simulink model "dof14model_rev"  (R2024a)
settings: Solver=ode4  StartTime=0.0  StopTime=simtime  FixedStep=samtime  RelTol=1e-3
values from neighbouring files (symbols this model uses):
  a = data(n,2)    [main_dof14model.m]
  b = data(n,3)    [main_dof14model.m]
  Csfl = data(n,22)    [main_dof14model.m]
  Csfr = data(n,23)    [main_dof14model.m]
  Csrl = data(n,24)    [main_dof14model.m]
  Csrr = data(n,25)    [main_dof14model.m]
  h = data(n,6)    [main_dof14model.m]
  Ip = data(n,10)    [main_dof14model.m]
  Ir = data(n,11)    [main_dof14model.m]
  Iw = data(n,17)    [main_dof14model.m]
  Jz = data(n,12)    [main_dof14model.m]
  Ksfl = data(n,18)    [main_dof14model.m]
  Ksfr = data(n,19)    [main_dof14model.m]
  Ksrl = data(n,20)    [main_dof14model.m]
  Ksrr = data(n,21)    [main_dof14model.m]
  Ktfl = data(n,28)    [main_dof14model.m]
  Ktfr = data(n,29)    [main_dof14model.m]
  Ktrl = data(n,30)    [main_dof14model.m]
  Ktrr = data(n,31)    [main_dof14model.m]
  Lf = data(n,8)    [main_dof14model.m]
  Lr = data(n,9)    [main_dof14model.m]
  Ms = data(n,1)    [main_dof14model.m]
  mt = data(n,7)    [main_dof14model.m]
  mufl = data(n,13)    [main_dof14model.m]
  mufr = data(n,14)    [main_dof14model.m]
  murl = data(n,15)    [main_dof14model.m]
  murr = data(n,16)    [main_dof14model.m]
  Rw = data(n,27)    [main_dof14model.m]
  wf = data(n,4)    [main_dof14model.m]
  wr = data(n,5)    [main_dof14model.m]
undefined symbols (not defined in the file or in its folder): sigbuilder_block
(part 1 of 2)
settings Model: Creator="Amrik  Singh"  LastModifiedBy=dltkd
settings SolverCC: ZeroCrossAlgorithm=Non-adaptive  AlgebraicLoopSolver=TrustRegion
settings DataIOCC: LimitDataPoints=on  SaveFormat=Array  SignalLoggingSaveFormat=ModelDataLogs  ReturnWorkspaceOutputs=off
settings OptimizationCC: ExpressionDepthLimit=2147483647  InitFltsAndDblsToZero=on  LifeSpan=inf
settings DebuggingCC: UnderspecifiedInitializationDetection=Classic  MergeDetectMultiDrivingBlocksExec=none  SolverPrmCheckMsg=warning  FcnCallInpInsideContextMsg=warning  UnconnectedInputMsg=warning  UnconnectedOutputMsg=warning  UnconnectedLineMsg=warning  StateNameClashWarn=warning  SFUnexpectedBacktrackingDiag=warning  SFNoUnconditionalDefaultTransitionDiag=warning  SFExecutionAtInitializationDiag=none  ArithmeticOperatorsInVariantConditions=warning
settings HardwareCC: ProdBitPerPointer=32  ProdBitPerSizeT=32  ProdBitPerPtrDiffT=32  ProdLargestAtomicFloat=None  ProdIntDivRoundTo=Undefined  ProdEndianess=Unspecified  ProdWordSize=32  ProdHWDeviceType=32-bit Generic
settings ModelReferenceCC: PropagateSignalLabelsOutOfModel=off
settings RTWCC: GPUComputeCapability=3.5
settings CodeAppCC: StateflowObjectComments=on
settings GRTTargetCC: TargetLangStandard=C89/C90 (ANSI)  CombineOutputUpdateFcns=off  GRTInterface=on
settings ConfigComp: CovMetricSettings=dw  CovSaveCumulativeToWorkspaceVar=on  CovSaveSingleToWorkspaceVar=on

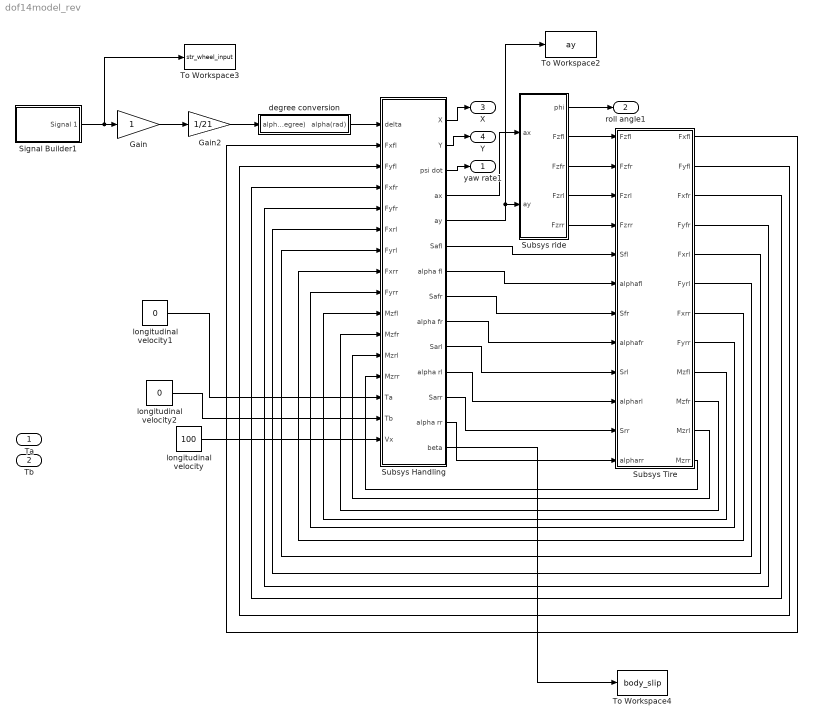
== system dof14model_rev ==
  Ta : Inport
  Tb : Inport  Port=2
  Gain : Gain
  Gain2 : Gain  Gain=1/21
  Signal Builder1 : Subsystem  Tag=STV Subsys  LoadFcn=sigbuilder_block('load');  StartFcn=sigbuilder_block('start');  StopFcn=sigbuilder_block('stop');  ClipboardFcn=sigbuilder_block('clipboard');  mask(Sigbuilder block){tuvar=[0:10]}
      mask help: Sigbuilder GUI
      mask init:
      | if ~strcmp(get_param(bdroot(gcbh),'SimulationStatus'),'stopped') tuvar = sigbuilder_block('maskInit'); end
      settings: CopyFcn=sigbuilder_block('copy');  DeleteFcn=sigbuilder_block('delete');  ModelCloseFcn=sigbuilder_block('modelClose');  PreSaveFcn=sigbuilder_block('preSave');  PauseFcn=sigbuilder_block('pause')  ContinueFcn=sigbuilder_block('continue')  NameChangeFcn=sigbuilder_block('namechange');  OpenFcn=sigbuilder_block('open',[214.5 118.2 550.5 399 ]);  CloseFcn=sigbuilder_block('close');
      mask Display: plot(0, 0, 100, 100,[2, 2, 32, 32, 2], [68, 8, 8, 68, 68],[32, 2], [38, 38], [32, 19, 2],[53, 60, 44], [32, 17, 17, 2],[16, 16, 31, 31]);txt = getActiveGroup(gcbh);text(2, 100, txt,'verticalAlignment', 'top');
  Subsys Handling : Subsystem
  Subsys Tire : Subsystem
  Subsys ride : Subsystem
  To Workspace2 : ToWorkspace  VariableName=ay  SampleTime=-1
      settings: Save2DSignal=2-D array (concatenate along first dimension)
  To Workspace3 : ToWorkspace  VariableName=str_wheel_input  SampleTime=-1
      settings: Save2DSignal=2-D array (concatenate along first dimension)
  To Workspace4 : ToWorkspace  VariableName=body_slip  SampleTime=-1
      settings: Save2DSignal=2-D array (concatenate along first dimension)
  degree conversion : Subsystem
  longitudinal velocity : Constant  Value=100
  longitudinal velocity1 : Constant  Value=0
  longitudinal velocity2 : Constant  Value=0
  yaw rate1 : Outport
  roll angle1 : Outport  Port=2
  X : Outport  Port=3
  Y : Outport  Port=4
  wires:
  Signal Builder1/1(Signal 1) -> To Workspace3/1, Gain/1
  Subsys Handling/2(Y) -> Y/1
  Subsys Tire/5(Fxrl) -> Subsys Handling/6(Fxrl)
  Subsys Handling/1(X) -> X/1
  Subsys Tire/7(Fxrr) -> Subsys Handling/8(Fxrr)
  Subsys ride/3(Fzfr) -> Subsys Tire/2(Fzfr)
  Subsys Tire/4(Fyfr) -> Subsys Handling/5(Fyfr)
  Subsys Handling/5(ay) -> To Workspace2/1, Subsys ride/2(ay)
  Subsys Tire/3(Fxfr) -> Subsys Handling/4(Fxfr)
  Subsys Tire/11(Mzrl) -> Subsys Handling/12(Mzrl)
  Subsys ride/1(phi) -> roll angle1/1
  Subsys ride/2(Fzfl) -> Subsys Tire/1(Fzfl)
  Subsys Tire/12(Mzrr) -> Subsys Handling/13(Mzrr)
  Subsys Tire/6(Fyrl) -> Subsys Handling/7(Fyrl)
  Subsys Handling/11(alpha rl) -> Subsys Tire/10(alpharl)
  Subsys Tire/9(Mzfl) -> Subsys Handling/10(Mzfl)
  Subsys Tire/1(Fxfl) -> Subsys Handling/2(Fxfl)
  Subsys Tire/10(Mzfr) -> Subsys Handling/11(Mzfr)
  Gain2/1 -> degree conversion/1(alpha(degree))
  Subsys Handling/3(psi dot) -> yaw rate1/1
  Subsys ride/5(Fzrr) -> Subsys Tire/4(Fzrr)
  Subsys Handling/6(Safl) -> Subsys Tire/5(Sfl)
  Subsys Tire/2(Fyfl) -> Subsys Handling/3(Fyfl)
  Subsys Handling/13(alpha rr) -> Subsys Tire/12(alpharr)
  Subsys Handling/10(Sarl) -> Subsys Tire/9(Srl)
  Subsys Tire/8(Fyrr) -> Subsys Handling/9(Fyrr)
  longitudinal velocity/1 -> Subsys Handling/16(Vx)
  Gain/1 -> Gain2/1
  Subsys Handling/9(alpha fr) -> Subsys Tire/8(alphafr)
  Subsys Handling/4(ax) -> Subsys ride/1(ax)
  Subsys Handling/8(Safr) -> Subsys Tire/7(Sfr)
  Subsys Handling/12(Sarr) -> Subsys Tire/11(Srr)
  Subsys Handling/7(alpha fl) -> Subsys Tire/6(alphafl)
  Subsys ride/4(Fzrl) -> Subsys Tire/3(Fzrl)
  degree conversion/1(alpha(rad)) -> Subsys Handling/1(delta)
  Subsys Handling/14(beta) -> To Workspace4/1
  longitudinal velocity1/1 -> Subsys Handling/14(Ta)
  longitudinal velocity2/1 -> Subsys Handling/15(Tb)

== system dof14model_rev/Signal Builder1 ==
  Demux : Demux  Tag=STV Demux  Outputs=1
      settings: DisplayOption=none
  FromWs : FromWorkspace  Tag=STV FromWs  VariableName=tuvar
      SigBuilderData=|
      | common.afterFinalStr = 'Extrapolate'
      | common.sampleTime = 0
      | dataSet.timeRange = [0 31]
      | dataSet.name = 'Group 1'
      | sbobj.Name = 'Signal Builder'
      | sbobj.Groups.Name = 'Group 1'
      | sbobj.Groups.Signals.Name = 'Signal 1'
      | sbobj.Groups.Signals.XData = [0 1 31]
      | sbobj.Groups.Signals.YData = [0 0 150]
      | sbobj.Groups.TimeRange = [0 31]
  Signal 1 : Outport  Tag=STV Outport
  wires:
  FromWs/1 -> Demux/1
  Demux/1 -> Signal 1/1

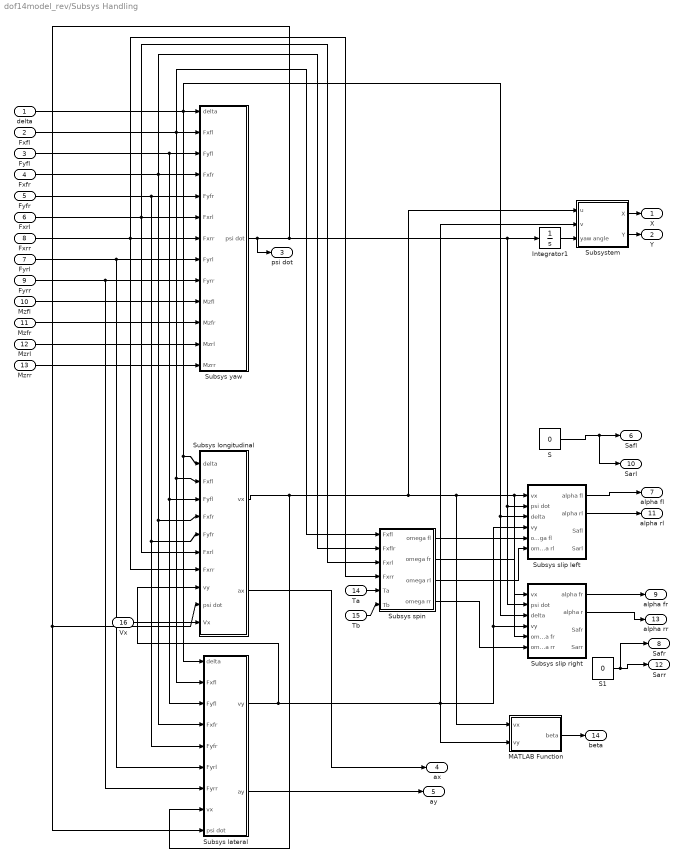
== system dof14model_rev/Subsys Handling ==
  delta : Inport
  Fxfl : Inport  Port=2
  Fyfl : Inport  Port=3
  Fxfr : Inport  Port=4
  Fyfr : Inport  Port=5
  Fxrl : Inport  Port=6
  Fyrl : Inport  Port=7
  Fxrr : Inport  Port=8
  Fyrr : Inport  Port=9
  Mzfl : Inport  Port=10
  Mzfr : Inport  Port=11
  Mzrl : Inport  Port=12
  Mzrr : Inport  Port=13
  Ta : Inport  Port=14
  Tb : Inport  Port=15
  Vx : Inport  Port=16
  Integrator1 : Integrator
  MATLAB Function : MATLAB Function  TreatAsAtomicUnit=on
  S : Constant  Value=0
  S1 : Constant  Value=0
  Subsys lateral : Subsystem
  Subsys longitudinal : Subsystem
  "Subsys slip left " : Subsystem
  Subsys slip right : Subsystem
  Subsys spin : Subsystem
  "Subsys yaw " : Subsystem
  Subsystem : Subsystem
  X : Outport
  Y : Outport  Port=2
  psi dot : Outport  Port=3
  ax : Outport  Port=4
  ay : Outport  Port=5
  Safl : Outport  Port=6
  alpha fl : Outport  Port=7
  Safr : Outport  Port=8
  alpha fr : Outport  Port=9
  Sarl : Outport  Port=10
  alpha rl : Outport  Port=11
  Sarr : Outport  Port=12
  alpha rr : Outport  Port=13
  beta : Outport  Port=14
  wires:
  Subsys lateral/2(ay) -> ay/1
  Subsys longitudinal/2(ax) -> ax/1
  Ta/1 -> Subsys spin/5(Ta)
  Tb/1 -> Subsys spin/6(Tb)
  "Subsys slip left "/1(alpha fl) -> alpha fl/1
  Subsys slip right/1(alpha fr) -> alpha fr/1
  Subsys slip right/2(alpha r) -> alpha rr/1
  Subsys spin/1(omega fl) -> "Subsys slip left "/5(omega fl)
  Subsys spin/4(omega rr) -> Subsys slip right/6(omega rr)
  Subsys longitudinal/1(vx) -> Subsys lateral/8(vx), MATLAB Function/1(vx), "Subsys slip left "/1(vx), Subsys slip right/1(vx), Subsystem/1(u)
  "Subsys slip left "/2(alpha rl) -> alpha rl/1
  delta/1 -> "Subsys yaw "/1(delta), Subsys longitudinal/1(delta), Subsys lateral/1(delta), "Subsys slip left "/3(delta), Subsys slip right/3(delta)
  Fxfl/1 -> "Subsys yaw "/2(Fxfl), Subsys longitudinal/2(Fxfl), Subsys lateral/2(Fxfl), Subsys spin/1(Fxfl)
  Fyfl/1 -> "Subsys yaw "/3(Fyfl), Subsys longitudinal/3(Fyfl), Subsys lateral/3(Fyfl)
  Fxfr/1 -> "Subsys yaw "/4(Fxfr), Subsys longitudinal/4(Fxfr), Subsys lateral/4(Fxfr), Subsys spin/2(Fxflr)
  Fyfr/1 -> "Subsys yaw "/5(Fyfr), Subsys longitudinal/5(Fyfr), Subsys lateral/5(Fyfr)
  Fxrl/1 -> "Subsys yaw "/6(Fxrl), Subsys spin/3(Fxrl), Subsys longitudinal/6(Fxrl)
  Fxrr/1 -> "Subsys yaw "/7(Fxrr), Subsys longitudinal/7(Fxrr), Subsys spin/4(Fxrr)
  Fyrl/1 -> "Subsys yaw "/8(Fyrl), Subsys lateral/6(Fyrl)
  Fyrr/1 -> "Subsys yaw "/9(Fyrr), Subsys lateral/7(Fyrr)
  "Subsys yaw "/1(psi dot) -> Subsys lateral/9("psi dot "), Subsys longitudinal/9("psi dot "), "Subsys slip left "/2(psi dot), Subsys slip right/2(psi dot), Integrator1/1, psi dot/1
  Subsys lateral/1(vy) -> Subsys longitudinal/8(vy), MATLAB Function/2(vy), "Subsys slip left "/4(vy), Subsys slip right/4(vy), Subsystem/2(v)
  Mzfl/1 -> "Subsys yaw "/10(Mzfl)
  Mzrr/1 -> "Subsys yaw "/13(Mzrr)
  Mzrl/1 -> "Subsys yaw "/12(Mzrl)
  Mzfr/1 -> "Subsys yaw "/11(Mzfr)
  Subsys spin/2(omega fr) -> Subsys slip right/5(omega fr)
  Subsys spin/3(omega rl) -> "Subsys slip left "/6(omega rl)
  S/1 -> Safl/1, Sarl/1
  S1/1 -> Sarr/1, Safr/1
  Vx/1 -> Subsys longitudinal/10(Vx)
  Integrator1/1 -> Subsystem/3(yaw angle)
  Subsystem/1(X) -> X/1
  Subsystem/2(Y) -> Y/1
  MATLAB Function/1(beta) -> beta/1

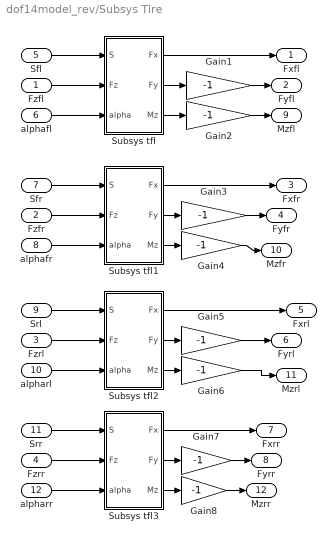
== system dof14model_rev/Subsys Tire ==
  Fzfl : Inport
  Fzfr : Inport  Port=2
  Fzrl : Inport  Port=3
  Fzrr : Inport  Port=4
  Sfl : Inport  Port=5
  alphafl : Inport  Port=6
  Sfr : Inport  Port=7
  alphafr : Inport  Port=8
  Srl : Inport  Port=9
  alpharl : Inport  Port=10
  Srr : Inport  Port=11
  alpharr : Inport  Port=12
  Gain{1..8} (8 alike) : Gain  Gain=-1
  Subsys tfl : Subsystem
  Subsys tfl1 : Subsystem
  Subsys tfl2 : Subsystem
  Subsys tfl3 : Subsystem
  Fxfl : Outport
  Fyfl : Outport  Port=2
  Fxfr : Outport  Port=3
  Fyfr : Outport  Port=4
  Fxrl : Outport  Port=5
  Fyrl : Outport  Port=6
  Fxrr : Outport  Port=7
  Fyrr : Outport  Port=8
  Mzfl : Outport  Port=9
  Mzfr : Outport  Port=10
  Mzrl : Outport  Port=11
  Mzrr : Outport  Port=12
  wires:
  Subsys tfl/1(Fx) -> Fxfl/1
  Subsys tfl/2(Fy) -> Gain1/1
  Subsys tfl/3(Mz) -> Gain2/1
  Sfl/1 -> Subsys tfl/1(S)
  Fzfl/1 -> Subsys tfl/2(Fz)
  alphafl/1 -> Subsys tfl/3(alpha)
  Subsys tfl1/1(Fx) -> Fxfr/1
  Subsys tfl1/2(Fy) -> Gain3/1
  Subsys tfl1/3(Mz) -> Gain4/1
  Sfr/1 -> Subsys tfl1/1(S)
  Fzfr/1 -> Subsys tfl1/2(Fz)
  alphafr/1 -> Subsys tfl1/3(alpha)
  Subsys tfl2/1(Fx) -> Fxrl/1
  Subsys tfl2/2(Fy) -> Gain5/1
  Subsys tfl2/3(Mz) -> Gain6/1
  Srl/1 -> Subsys tfl2/1(S)
  Fzrl/1 -> Subsys tfl2/2(Fz)
  alpharl/1 -> Subsys tfl2/3(alpha)
  Subsys tfl3/1(Fx) -> Fxrr/1
  Subsys tfl3/2(Fy) -> Gain7/1
  Subsys tfl3/3(Mz) -> Gain8/1
  Srr/1 -> Subsys tfl3/1(S)
  Fzrr/1 -> Subsys tfl3/2(Fz)
  alpharr/1 -> Subsys tfl3/3(alpha)
  Gain1/1 -> Fyfl/1
  Gain2/1 -> Mzfl/1
  Gain3/1 -> Fyfr/1
  Gain4/1 -> Mzfr/1
  Gain5/1 -> Fyrl/1
  Gain6/1 -> Mzrl/1
  Gain7/1 -> Fyrr/1
  Gain8/1 -> Mzrr/1

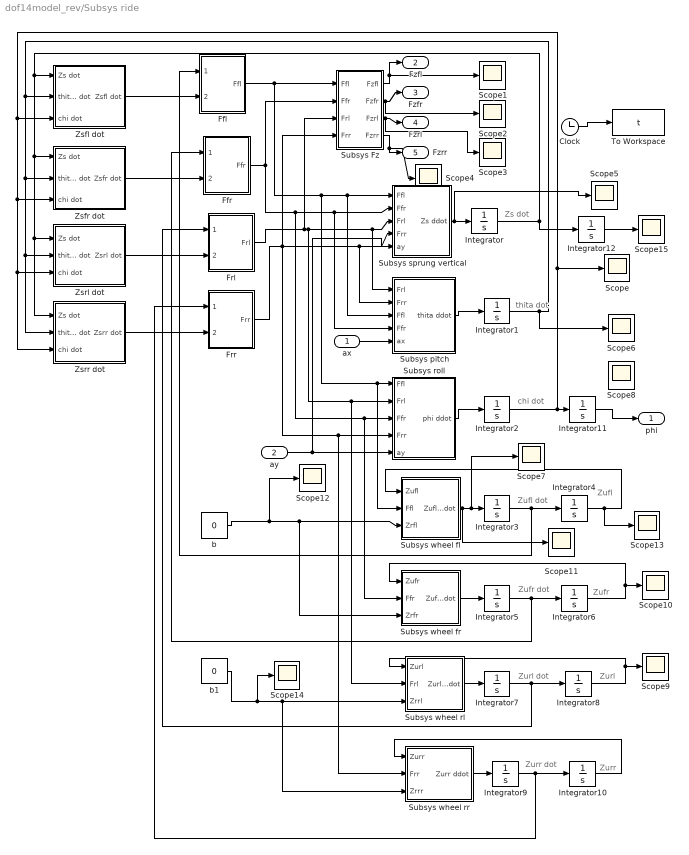
== system dof14model_rev/Subsys ride ==
  note: Zs dot
  note: thita dot
  note: chi dot
  note: Zufl dot
  note: Zufr dot
  note: Zurl dot
  note: Zurr dot
  note: Zufl
  note: Zufr
  note: Zurl
  note: Zurr
  ax : Inport
  ay : Inport  Port=2
  Clock : Clock
  Ffl : Subsystem
  Ffr : Subsystem
  Frl : Subsystem
  Frr : Subsystem
  Integrator{,1..12} (13 alike) : Integrator
  Scope{,1..15} (16 alike) : Scope
  Subsys Fz : Subsystem
  Subsys pitch : Subsystem
  Subsys roll : Subsystem
  Subsys sprung vertical : Subsystem
  Subsys wheel fl : Subsystem
  Subsys wheel fr : Subsystem
  Subsys wheel rl : Subsystem
  Subsys wheel rr : Subsystem
  To Workspace : ToWorkspace  VariableName=t  SampleTime=-1
  Zsfl dot : Subsystem
  Zsfr dot : Subsystem
  Zsrl dot : Subsystem
  Zsrr dot : Subsystem
  b : Constant  Value=0
  b1 : Constant  Value=0
  phi : Outport
  Fzfl : Outport  Port=2
  Fzfr : Outport  Port=3
  Fzrl : Outport  Port=4
  Fzrr : Outport  Port=5
  wires:
  Ffl/1(Ffl) -> Subsys sprung vertical/1(Ffl), Subsys pitch/3(Ffl), Subsys wheel fl/2(Ffl), Subsys roll/1(Ffl), Subsys Fz/1(Ffl)
  Ffr/1(Ffr) -> Subsys sprung vertical/2(Ffr), Subsys pitch/4(Ffr), Subsys wheel fr/2(Ffr), Subsys roll/3(Ffr), Subsys Fz/2(Ffr)
  Frl/1(Frl) -> Subsys sprung vertical/3(Frl), Subsys pitch/1(Frl), Subsys wheel rl/2(Frl), Subsys roll/2(Frl), Subsys Fz/3(Frl)
  Frr/1(Frr) -> Subsys sprung vertical/4(Frr), Subsys pitch/2(Frr), Subsys wheel rr/2(Frr), Subsys roll/4(Frr), Subsys Fz/4(Frr)
  Subsys sprung vertical/1(Zs ddot) -> Integrator/1, Scope5/1
  Integrator/1 -> Zsrr dot/1(Zs dot), Zsrl dot/1(Zs dot), Zsfr dot/1(Zs dot), Zsfl dot/1(Zs dot), Integrator12/1
  Zsfr dot/1(Zsfr dot) -> Ffr/2(Zsfr dot)
  Zsfl dot/1(Zsfl dot) -> Ffl/2(Zsfl dot)
  Zsrl dot/1(Zsrl dot) -> Frl/2(Zsrl dot)
  Zsrr dot/1(Zsrr dot) -> Frr/2(Zsrr dot)
  Subsys pitch/1(thita ddot) -> Integrator1/1
  Subsys roll/1(phi ddot) -> Integrator2/1
  Integrator2/1 -> Zsrr dot/3(chi dot), Zsrl dot/3(chi dot), Zsfr dot/3(chi dot), Zsfl dot/3(chi dot), Scope/1, Integrator11/1
  Subsys wheel fl/1(Zufl ddot) -> Integrator3/1, Scope7/1, Scope11/1
  Integrator3/1 -> Integrator4/1, Ffl/1(Zufl dot)
  Subsys wheel fr/1(Zufr ddot) -> Integrator5/1
  Integrator5/1 -> Integrator6/1, Ffr/1(Zufr dot)
  Subsys wheel rl/1(Zurl ddot) -> Integrator7/1
  Integrator7/1 -> Integrator8/1, Frl/1(Zurl dot)
  Subsys wheel rr/1(Zurr ddot) -> Integrator9/1
  Integrator9/1 -> Integrator10/1, Frr/1(Zurr dot)
  Integrator4/1 -> Subsys wheel fl/1(Zufl), Scope13/1
  Integrator6/1 -> Subsys wheel fr/1(Zufr), Scope10/1
  Integrator8/1 -> Scope9/1, Subsys wheel rl/1(Zurl)
  Integrator10/1 -> Subsys wheel rr/1(Zurr)
  Clock/1 -> To Workspace/1
  Integrator1/1 -> Zsrr dot/2(thita dot), Zsrl dot/2(thita dot), Zsfr dot/2(thita dot), Zsfl dot/2(thita dot), Scope6/1
  Subsys Fz/1(Fzfl) -> Fzfl/1, Scope1/1
  Subsys Fz/2(Fzfr) -> Fzfr/1, Scope2/1
  Subsys Fz/3(Fzrl) -> Fzrl/1, Scope3/1
  Subsys Fz/4(Fzrr) -> Fzrr/1, Scope4/1
  b/1 -> Subsys wheel fl/3(Zrfl), Subsys wheel fr/3(Zrfr), Scope12/1
  b1/1 -> Subsys wheel rl/3(Zrrl), Subsys wheel rr/3(Zrrr), Scope14/1
  ay/1 -> Subsys roll/5(ay), Subsys sprung vertical/5(ay)
  ax/1 -> Subsys pitch/5(ax)
  Integrator11/1 -> phi/1
  Integrator12/1 -> Scope15/1

== system dof14model_rev/degree conversion ==
  alpha(degree) : Inport
  180 degrees : Constant  Value=180
  Divide : Product  Inputs=**/
  pi : Constant  Value=22/7
  alpha(rad) : Outport
  wires:
  alpha(degree)/1 -> Divide/1
  Divide/1 -> alpha(rad)/1
  pi/1 -> Divide/2
  180 degrees/1 -> Divide/3

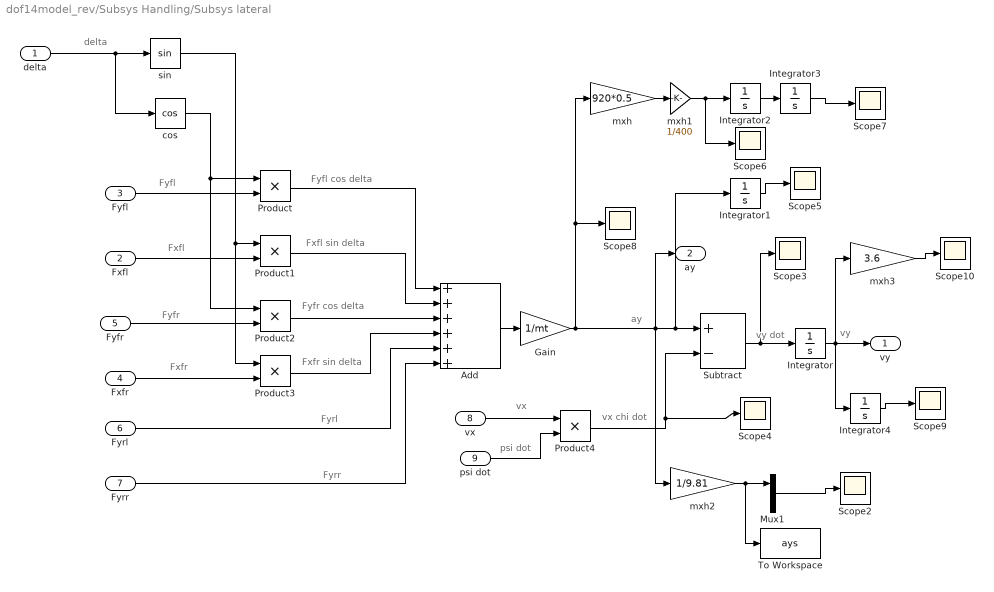
== system dof14model_rev/Subsys Handling/Subsys lateral ==
  note: vy
  note: vy dot
  note: ay
  note: vx
  note: delta
  note: Fyrr
  note: Fyrl
  note: Fxfr
  note: Fyfr
  note: Fxfl
  note: Fyfl
  note: Fyfl cos delta
  note: Fxfl sin delta
  note: Fyfr cos delta
  note: Fxfr sin delta
  note: vx chi dot
  note: psi dot
  delta : Inport
  Fxfl : Inport  Port=2
  Fyfl : Inport  Port=3
  Fxfr : Inport  Port=4
  Fyfr : Inport  Port=5
  Fyrl : Inport  Port=6
  Fyrr : Inport  Port=7
  vx : Inport  Port=8
  "psi dot " : Inport  Port=9
  Add : Sum  Inputs=++++++
  Gain : Gain  Gain=1/mt
  Integrator{,1..4} (5 alike) : Integrator
  Mux1 : Mux  Inputs=2
  Product{,1..4} (5 alike) : Product  RndMeth=Zero
  Scope{2..10} (9 alike) : Scope
  Subtract : Sum  Inputs=+-
  To Workspace : ToWorkspace  VariableName=ays  SampleTime=-1
  cos : Trigonometry  Operator=cos
  mxh : Gain  Gain=920*0.5
  mxh1 : Gain  Gain=1/400
  mxh2 : Gain  Gain=1/9.81
  mxh3 : Gain  Gain=3.6
  sin : Trigonometry
  vy : Outport
  ay : Outport  Port=2
  wires:
  Integrator/1 -> vy/1, Integrator4/1, mxh3/1
  Subtract/1 -> Integrator/1, Scope3/1
  Product4/1 -> Subtract/2, Scope4/1
  Gain/1 -> ay/1, Subtract/1, Integrator1/1, mxh2/1, mxh/1, Scope8/1
  vx/1 -> Product4/1
  Add/1 -> Gain/1
  Fyrr/1 -> Add/6
  Fyrl/1 -> Add/5
  Product3/1 -> Add/4
  Product2/1 -> Add/3
  Product1/1 -> Add/2
  Product/1 -> Add/1
  Fxfr/1 -> Product3/2
  Fyfr/1 -> Product2/2
  Fxfl/1 -> Product1/2
  Fyfl/1 -> Product/2
  sin/1 -> Product1/1, Product3/1
  cos/1 -> Product2/1, Product/1
  delta/1 -> cos/1, sin/1
  Integrator1/1 -> Scope5/1
  "psi dot "/1 -> Product4/2
  Mux1/1 -> Scope2/1
  mxh/1 -> mxh1/1
  Integrator2/1 -> Integrator3/1
  Integrator3/1 -> Scope7/1
  mxh1/1 -> Scope6/1, Integrator2/1
  Integrator4/1 -> Scope9/1
  mxh2/1 -> Mux1/1, To Workspace/1
  mxh3/1 -> Scope10/1

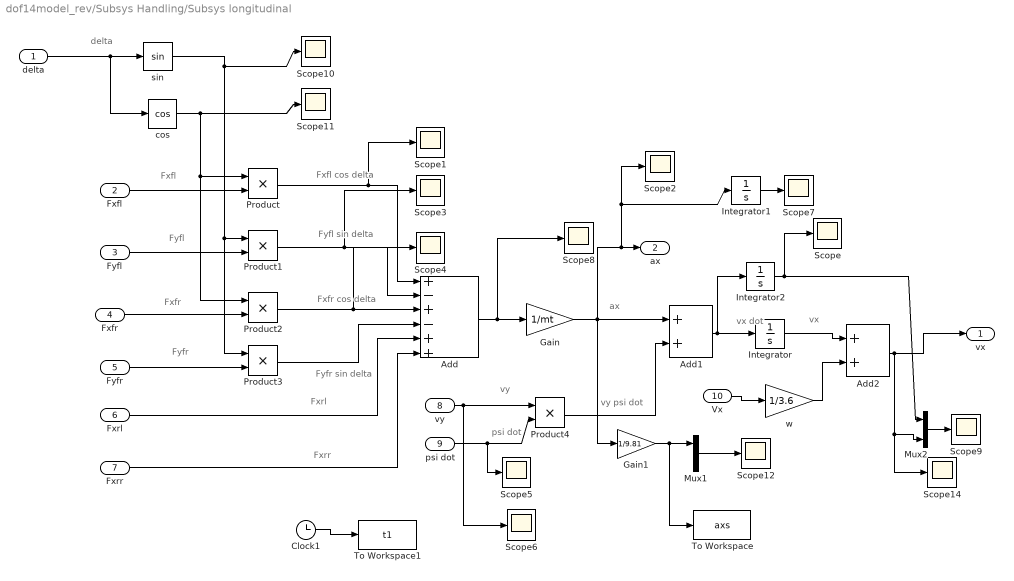
== system dof14model_rev/Subsys Handling/Subsys longitudinal ==
  note: Fxfl
  note: Fyfl
  note: Fxfr
  note: Fyfr
  note: Fxrl
  note: Fxrr
  note: delta
  note: vy
  note: ax
  note: vx dot
  note: vx
  note: Fxfl cos delta
  note: Fyfl sin delta
  note: Fxfr cos delta
  note: Fyfr sin delta
  note: psi dot
  note: vy psi dot
  delta : Inport
  Fxfl : Inport  Port=2
  Fyfl : Inport  Port=3
  Fxfr : Inport  Port=4
  Fyfr : Inport  Port=5
  Fxrl : Inport  Port=6
  Fxrr : Inport  Port=7
  vy : Inport  Port=8
  "psi dot " : Inport  Port=9
  Vx : Inport  Port=10
  Add : Sum  Inputs=+-+-++
  Add1 : Sum
  Add2 : Sum
  Clock1 : Clock
  Gain : Gain  Gain=1/mt
  Gain1 : Gain  Gain=1/9.81
  Integrator : Integrator
  Integrator1 : Integrator
  Integrator2 : Integrator  InitialCondition=50/3.6
  Mux1 : Mux  Inputs=2
  Mux2 : Mux  Inputs=2
  Product{,1..4} (5 alike) : Product  RndMeth=Zero
  Scope{,1..12,14} (14 alike) : Scope
  To Workspace : ToWorkspace  VariableName=axs  SampleTime=-1
  To Workspace1 : ToWorkspace  VariableName=t1  SampleTime=-1
  cos : Trigonometry  Operator=cos
  sin : Trigonometry
  w : Gain  Gain=1/3.6
  vx : Outport
  ax : Outport  Port=2
  wires:
  delta/1 -> sin/1, cos/1
  cos/1 -> Product/1, Product2/1, Scope11/1
  sin/1 -> Product3/1, Product1/1, Scope10/1
  Fxfl/1 -> Product/2
  Fyfl/1 -> Product1/2
  Fxfr/1 -> Product2/2
  Fyfr/1 -> Product3/2
  Product/1 -> Add/1, Scope1/1
  Product1/1 -> Add/2, Scope3/1
  Product2/1 -> Add/3, Scope4/1
  Product3/1 -> Add/4
  Fxrl/1 -> Add/5
  Fxrr/1 -> Add/6
  Add/1 -> Gain/1, Scope8/1
  "psi dot "/1 -> Product4/2, Scope5/1
  vy/1 -> Product4/1, Scope6/1
  Gain/1 -> ax/1, Scope2/1, Integrator1/1, Gain1/1, Add1/1
  Add1/1 -> Integrator/1, Integrator2/1
  Integrator/1 -> Add2/1
  Product4/1 -> Add1/2
  Integrator1/1 -> Scope7/1
  ? -> Mux1/2
  Mux1/1 -> Scope12/1
  Gain1/1 -> Mux1/1, To Workspace/1
  Clock1/1 -> To Workspace1/1
  w/1 -> Add2/2
  Add2/1 -> vx/1, Mux2/2, Scope14/1
  Vx/1 -> w/1
  Mux2/1 -> Scope9/1
  Integrator2/1 -> Mux2/1, Scope/1

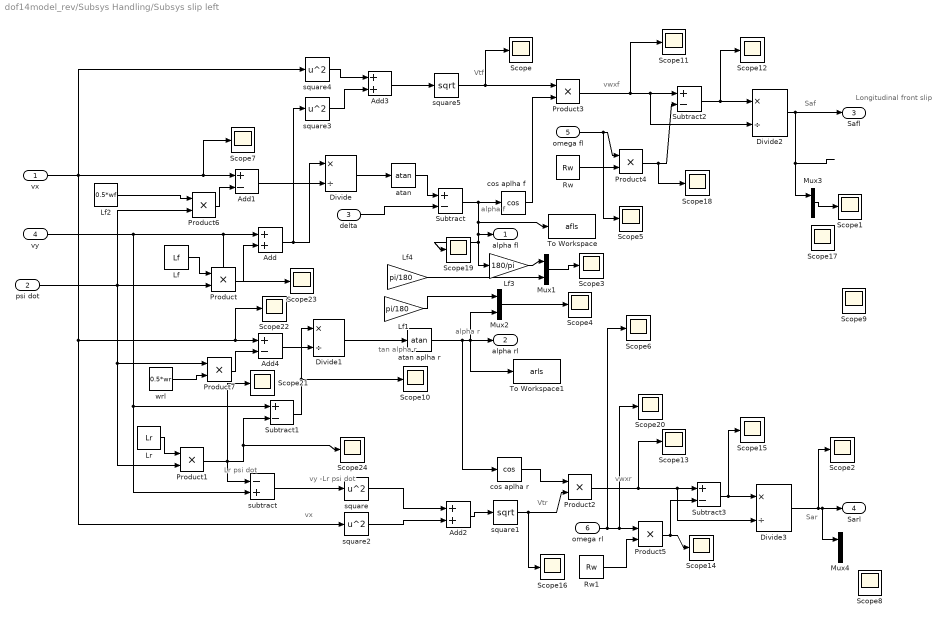
== system dof14model_rev/Subsys Handling/Subsys slip left  ==
  note: tan alpha r
  note: alpha r
  note: Lr psi dot
  note: vx
  note: vy -Lr psi dot
  note: Vtr
  note: alpha f
  note: vwxr
  note: Vtf
  note: vwxf
  note: Saf
  note: Longitudinal front slip
  note: Sar
  vx : Inport
  psi dot : Inport  Port=2
  delta : Inport  Port=3
  vy : Inport  Port=4
  omega fl : Inport  Port=5
  omega rl : Inport  Port=6
  Add : Sum
  Add1 : Sum  Inputs=+-
  Add2 : Sum
  Add3 : Sum
  Add4 : Sum  Inputs=+-
  Divide{,1..3} (4 alike) : Product  Inputs=*/
  Lf : Constant  Value=Lf
  Lf1 : Gain  Gain=pi/180
  Lf2 : Constant  Value=0.5*wf
  Lf3 : Gain  Gain=180/pi
  Lf4 : Gain  Gain=pi/180
  Lr : Constant  Value=Lr
  Mux{1..4} (4 alike) : Mux  Inputs=2
  Product{,1..7} (8 alike) : Product  RndMeth=Zero
  Rw : Constant  Value=Rw
  Rw1 : Constant  Value=Rw
  Scope{,1..24} (25 alike) : Scope
  Subtract{,1..3} (4 alike) : Sum  Inputs=+-
  To Workspace : ToWorkspace  VariableName=afls  SampleTime=-1
  To Workspace1 : ToWorkspace  VariableName=arls  SampleTime=-1
  "atan " : Trigonometry  Operator=atan
  atan aplha r : Trigonometry  Operator=atan
  cos aplha f : Trigonometry  Operator=cos
  cos aplha r : Trigonometry  Operator=cos
  square{,2..4} (4 alike) : Math  Operator=square  SignedPower=on
  square1 : Math  Operator=sqrt  SignedPower=on
  square5 : Math  Operator=sqrt  SignedPower=on
  subtract : Sum  Inputs=-+
  wrl : Constant  Value=0.5*wr
  alpha fl : Outport
  alpha rl : Outport  Port=2
  Safl : Outport  Port=3
  Sarl : Outport  Port=4
  wires:
  Lf/1 -> Product/1
  psi dot/1 -> Product/2, Product6/2, Product1/2, Product7/1
  Add/1 -> Divide/1, square3/1
  delta/1 -> Subtract/2
  vx/1 -> square4/1, Add1/1, Scope7/1, square2/1, Add4/1, Scope22/1
  Product/1 -> Add/2
  vy/1 -> Subtract1/1, subtract/2, Add/1, Scope23/1
  Divide/1 -> "atan "/1
  "atan "/1 -> Subtract/1
  Subtract1/1 -> Divide1/1, Scope10/1
  Lr/1 -> Product1/1
  Product1/1 -> subtract/1, Scope21/1, Subtract1/2, Scope24/1
  Divide1/1 -> atan aplha r/1
  atan aplha r/1 -> cos aplha r/1, alpha rl/1, Mux2/2, To Workspace1/1
  subtract/1 -> square/1
  square/1 -> Add2/1
  square2/1 -> Add2/2
  Add2/1 -> square1/1
  square1/1 -> Product2/2, Scope16/1
  cos aplha r/1 -> Product2/1
  Product2/1 -> Scope13/1, Subtract3/1, Divide3/2
  square4/1 -> Add3/1
  square3/1 -> Add3/2
  Add3/1 -> square5/1
  Subtract/1 -> cos aplha f/1, alpha fl/1, Lf3/1, Scope19/1, To Workspace/1
  square5/1 -> Product3/1, Scope/1
  cos aplha f/1 -> Product3/2
  Product3/1 -> Subtract2/1, Divide2/2, Scope11/1
  omega fl/1 -> Product4/1, Scope5/1
  Rw/1 -> Product4/2
  Product4/1 -> Subtract2/2, Scope18/1
  Subtract2/1 -> Divide2/1, Scope12/1
  Divide2/1 -> Safl/1, Mux3/1
  omega rl/1 -> Scope6/1, Product5/1, Scope20/1
  Rw1/1 -> Product5/2
  Product5/1 -> Scope14/1, Subtract3/2
  Subtract3/1 -> Divide3/1, Scope15/1
  Divide3/1 -> Sarl/1, Mux4/1, Scope2/1
  ? -> Lf4/1
  Mux1/1 -> Scope3/1
  Lf4/1 -> Mux1/2
  ? -> Lf1/1
  Mux2/1 -> Scope4/1
  Lf1/1 -> Mux2/1
  ? -> Mux3/2, Scope17/1
  Mux3/1 -> Scope1/1
  ? -> Scope9/1
  Add1/1 -> Divide/2
  Product6/1 -> Add1/2
  Lf2/1 -> Product6/1
  wrl/1 -> Product7/2
  Add4/1 -> Divide1/2
  Product7/1 -> Add4/2
  ? -> Scope8/1
  Lf3/1 -> Mux1/1

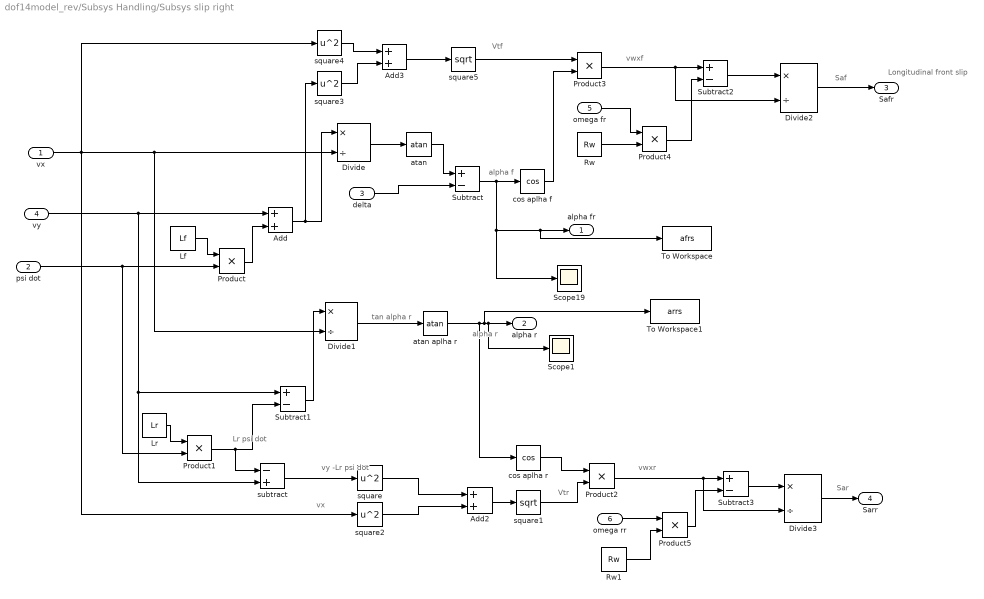
== system dof14model_rev/Subsys Handling/Subsys slip right ==
  note: Sar
  note: Longitudinal front slip
  note: Saf
  note: vwxf
  note: Vtf
  note: vwxr
  note: alpha f
  note: Vtr
  note: vy -Lr psi dot
  note: vx
  note: Lr psi dot
  note: alpha r
  note: tan alpha r
  vx : Inport
  psi dot : Inport  Port=2
  delta : Inport  Port=3
  vy : Inport  Port=4
  omega fr : Inport  Port=5
  omega rr : Inport  Port=6
  Add : Sum
  Add2 : Sum
  Add3 : Sum
  Divide{,1..3} (4 alike) : Product  Inputs=*/
  Lf : Constant  Value=Lf
  Lr : Constant  Value=Lr
  Product{,1..5} (6 alike) : Product  RndMeth=Zero
  Rw : Constant  Value=Rw
  Rw1 : Constant  Value=Rw
  Scope1 : Scope
  Scope19 : Scope
  Subtract{,1..3} (4 alike) : Sum  Inputs=+-
  To Workspace : ToWorkspace  VariableName=afrs  SampleTime=-1
  To Workspace1 : ToWorkspace  VariableName=arrs  SampleTime=-1
  "atan " : Trigonometry  Operator=atan
  atan aplha r : Trigonometry  Operator=atan
  cos aplha f : Trigonometry  Operator=cos
  cos aplha r : Trigonometry  Operator=cos
  square{,2..4} (4 alike) : Math  Operator=square  SignedPower=on
  square1 : Math  Operator=sqrt  SignedPower=on
  square5 : Math  Operator=sqrt  SignedPower=on
  subtract : Sum  Inputs=-+
  alpha fr : Outport
  alpha r : Outport  Port=2
  Safr : Outport  Port=3
  Sarr : Outport  Port=4
  wires:
  Divide3/1 -> Sarr/1
  Subtract3/1 -> Divide3/1
  Product5/1 -> Subtract3/2
  Rw1/1 -> Product5/2
  omega rr/1 -> Product5/1
  Divide2/1 -> Safr/1
  Subtract2/1 -> Divide2/1
  Product4/1 -> Subtract2/2
  Rw/1 -> Product4/2
  omega fr/1 -> Product4/1
  Product3/1 -> Divide2/2, Subtract2/1
  cos aplha f/1 -> Product3/2
  square5/1 -> Product3/1
  Subtract/1 -> cos aplha f/1, Scope19/1, alpha fr/1, To Workspace/1
  Add3/1 -> square5/1
  square3/1 -> Add3/2
  square4/1 -> Add3/1
  Product2/1 -> Divide3/2, Subtract3/1
  cos aplha r/1 -> Product2/1
  square1/1 -> Product2/2
  Add2/1 -> square1/1
  square2/1 -> Add2/2
  square/1 -> Add2/1
  subtract/1 -> square/1
  atan aplha r/1 -> cos aplha r/1, alpha r/1, Scope1/1, To Workspace1/1
  Divide1/1 -> atan aplha r/1
  Product1/1 -> subtract/1, Subtract1/2
  Lr/1 -> Product1/1
  Subtract1/1 -> Divide1/1
  "atan "/1 -> Subtract/1
  Divide/1 -> "atan "/1
  vy/1 -> subtract/2, Subtract1/1, Add/1
  Product/1 -> Add/2
  vx/1 -> square4/1, Divide1/2, Divide/2, square2/1
  delta/1 -> Subtract/2
  Add/1 -> square3/1, Divide/1
  psi dot/1 -> Product1/2, Product/2
  Lf/1 -> Product/1

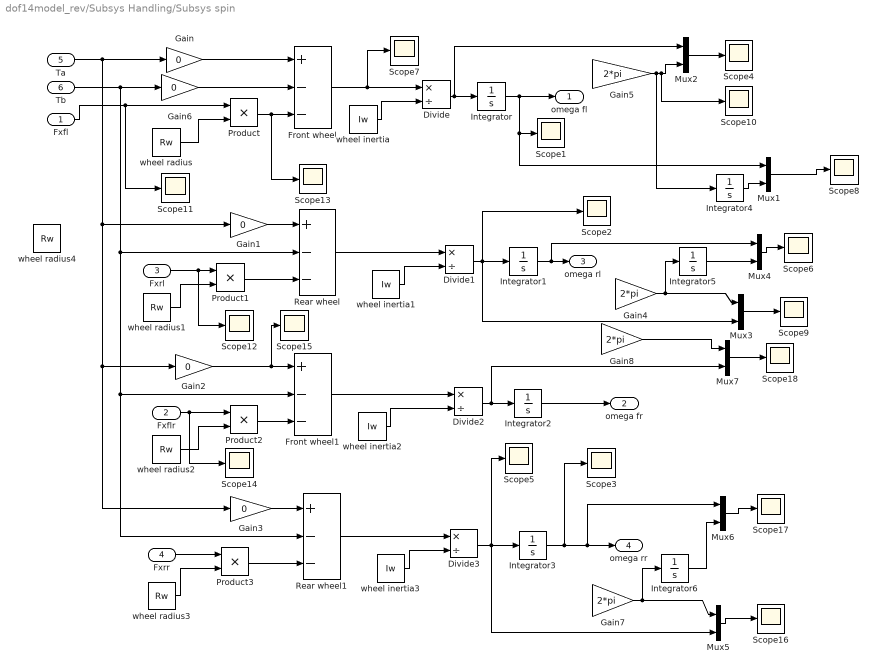
== system dof14model_rev/Subsys Handling/Subsys spin ==
  Fxfl : Inport
  Fxflr : Inport  Port=2
  Fxrl : Inport  Port=3
  Fxrr : Inport  Port=4
  Ta : Inport  Port=5
  Tb : Inport  Port=6
  Divide{,1..3} (4 alike) : Product  Inputs=*/
  Front wheel : Sum  Inputs=+--
  Front wheel1 : Sum  Inputs=+--
  Gain{,1..3,6} (5 alike) : Gain  Gain=0
  Gain{4..5,7..8} (4 alike) : Gain  Gain=2*pi
  Integrator{,1..6} (7 alike) : Integrator
  Mux{1..7} (7 alike) : Mux  Inputs=2
  Product{,1..3} (4 alike) : Product  RndMeth=Zero
  Rear wheel : Sum  Inputs=+--
  Rear wheel1 : Sum  Inputs=+--
  Scope{1..18} (18 alike) : Scope
  wheel inertia{,1..3} (4 alike) : Constant  Value=Iw
  wheel radius{,1..4} (5 alike) : Constant  Value=Rw
  omega fl : Outport
  omega fr : Outport  Port=2
  omega rl : Outport  Port=3
  omega rr : Outport  Port=4
  wires:
  Ta/1 -> Gain/1, Gain1/1, Gain2/1, Gain3/1
  Gain1/1 -> Rear wheel/1
  Gain/1 -> Front wheel/1
  Tb/1 -> Rear wheel/2, Front wheel1/2, Rear wheel1/2, Gain6/1
  Front wheel/1 -> Divide/1, Scope7/1
  Rear wheel/1 -> Divide1/1
  Product1/1 -> Rear wheel/3
  wheel inertia/1 -> Divide/2
  wheel inertia1/1 -> Divide1/2
  Divide/1 -> Integrator/1, Mux2/1
  Divide1/1 -> Integrator1/1, Scope2/1, Mux3/2
  Fxfl/1 -> Product/1, Scope11/1
  Product/1 -> Front wheel/3, Scope13/1
  wheel radius/1 -> Product/2
  Fxrl/1 -> Product1/1, Scope12/1
  wheel radius1/1 -> Product1/2
  Gain2/1 -> Front wheel1/1, Scope15/1
  Front wheel1/1 -> Divide2/1
  wheel inertia2/1 -> Divide2/2
  Fxflr/1 -> Product2/1, Scope14/1
  Product2/1 -> Front wheel1/3
  wheel radius2/1 -> Product2/2
  Gain3/1 -> Rear wheel1/1
  Rear wheel1/1 -> Divide3/1
  Product3/1 -> Rear wheel1/3
  wheel inertia3/1 -> Divide3/2
  Divide3/1 -> Integrator3/1, Scope5/1, Mux5/2
  Fxrr/1 -> Product3/1
  wheel radius3/1 -> Product3/2
  Integrator/1 -> omega fl/1, Scope1/1, Mux1/1
  Integrator1/1 -> omega rl/1, Mux4/1
  Divide2/1 -> Integrator2/1, Mux7/2
  Integrator2/1 -> omega fr/1
  Integrator3/1 -> Scope3/1, omega rr/1, Mux6/1
  Mux1/1 -> Scope8/1
  ? -> Gain5/1
  Gain5/1 -> Integrator4/1, Mux2/2, Scope10/1
  Mux2/1 -> Scope4/1
  Integrator4/1 -> Mux1/2
  Mux3/1 -> Scope9/1
  ? -> Gain4/1
  Gain4/1 -> Mux3/1, Integrator5/1
  Integrator5/1 -> Mux4/2
  Mux4/1 -> Scope6/1
  Gain6/1 -> Front wheel/2
  Mux5/1 -> Scope16/1
  ? -> Gain7/1
  Gain7/1 -> Mux5/1, Integrator6/1
  Integrator6/1 -> Mux6/2
  Mux6/1 -> Scope17/1
  Mux7/1 -> Scope18/1
  Gain8/1 -> Mux7/1
  ? -> Gain8/1

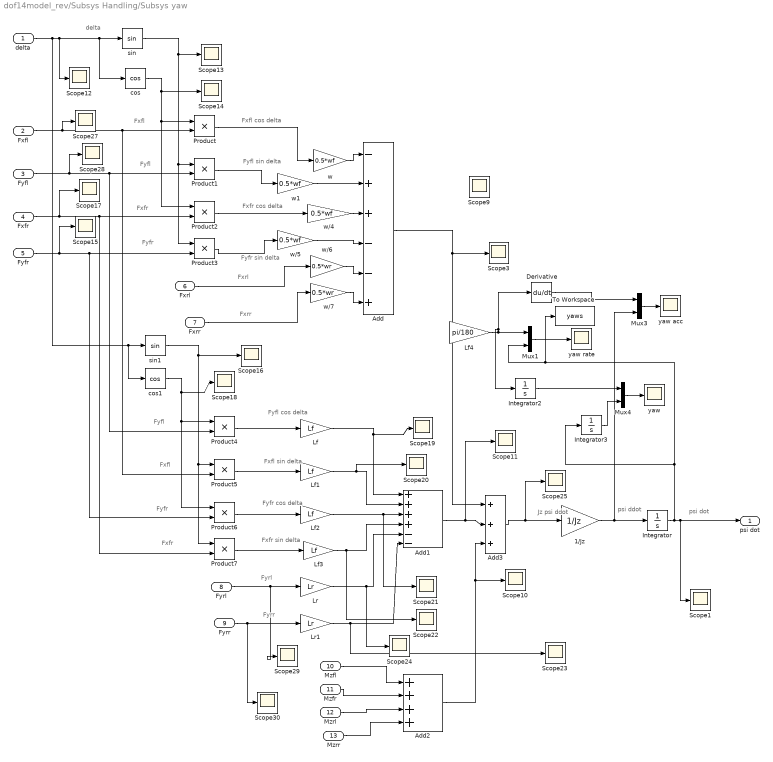
== system dof14model_rev/Subsys Handling/Subsys yaw  ==
  note: Fxfl
  note: Fyfl
  note: Fxfr
  note: Fyfr
  note: Fxrl
  note: Fxrr
  note: delta
  note: Fxfl cos delta
  note: Fyfl sin delta
  note: Fxfr cos delta
  note: Fyfr sin delta
  note: Fyrr
  note: Fyrl
  note: Fxfr
  note: Fyfr
  note: Fxfl
  note: Fyfl
  note: Fyfl cos delta
  note: Fxfl sin delta
  note: Fyfr cos delta
  note: Fxfr sin delta
  note: Jz psi ddot
  note: psi ddot
  note: psi dot
  delta : Inport
  Fxfl : Inport  Port=2
  Fyfl : Inport  Port=3
  Fxfr : Inport  Port=4
  Fyfr : Inport  Port=5
  Fxrl : Inport  Port=6
  Fxrr : Inport  Port=7
  Fyrl : Inport  Port=8
  Fyrr : Inport  Port=9
  Mzfl : Inport  Port=10
  Mzfr : Inport  Port=11
  Mzrl : Inport  Port=12
  Mzrr : Inport  Port=13
  1/Jz : Gain  Gain=1/Jz
  Add : Sum  Inputs=-++--+
  Add1 : Sum  Inputs=++++--
  Add2 : Sum  Inputs=++++
  Add3 : Sum  Inputs=+++
  Derivative : Derivative
  Integrator : Integrator
  Integrator2 : Integrator
  Integrator3 : Integrator
  Lf{,1..3} (4 alike) : Gain  Gain=Lf
  Lf4 : Gain  Gain=pi/180
  Lr : Gain  Gain=Lr
  Lr1 : Gain  Gain=Lr
  Mux1 : Mux  Inputs=2
  Mux3 : Mux  Inputs=2
  Mux4 : Mux  Inputs=2
  Product{,1..7} (8 alike) : Product  RndMeth=Zero
  Scope{1,3,9..25,27..30} (23 alike) : Scope
  To Workspace : ToWorkspace  VariableName=yaws  SampleTime=-1
  cos : Trigonometry  Operator=cos
  cos1 : Trigonometry  Operator=cos
  sin : Trigonometry
  sin1 : Trigonometry
  w : Gain  Gain=0.5*wf
  w/4 : Gain  Gain=0.5*wf
  w/5 : Gain  Gain=0.5*wf
  w/6 : Gain  Gain=0.5*wr
  w/7 : Gain  Gain=0.5*wr
  w1 : Gain  Gain=0.5*wf
  yaw : Scope
  yaw acc : Scope
  yaw rate : Scope
  psi dot : Outport
  wires:
  delta/1 -> sin1/1, cos1/1, sin/1, cos/1, Scope12/1
  cos/1 -> Product/1, Product2/1, Scope14/1
  sin/1 -> Product3/1, Product1/1, Scope13/1
  Fxfl/1 -> Product/2, Product5/2, Scope27/1
  Fyfl/1 -> Product1/2, Product4/2, Scope28/1
  Fxfr/1 -> Product2/2, Product7/2, Scope17/1
  Fyfr/1 -> Product3/2, Product6/2, Scope15/1
  Product2/1 -> w/4/1
  Product3/1 -> w/5/1
  Fxrl/1 -> w/6/1
  Fxrr/1 -> w/7/1
  Product1/1 -> w1/1
  Product/1 -> w/1
  sin1/1 -> Product5/1, Product7/1, Scope16/1
  cos1/1 -> Product6/1, Product4/1, Scope18/1
  Product4/1 -> Lf/1
  Lf/1 -> Add1/1, Scope19/1
  Product5/1 -> Lf1/1
  Product6/1 -> Lf2/1
  Product7/1 -> Lf3/1
  Lf1/1 -> Add1/2, Scope20/1
  Lf2/1 -> Add1/3, Scope21/1
  Lf3/1 -> Add1/4, Scope22/1
  Fyrr/1 -> Lr1/1, Scope30/1
  Lr/1 -> Add1/5, Scope24/1
  Lr1/1 -> Add1/6, Scope23/1
  Add/1 -> Add3/1, Scope3/1
  Fyrl/1 -> Lr/1, Scope29/1
  Integrator/1 -> Integrator3/1, Mux1/2, To Workspace/1, Scope1/1, psi dot/1
  1/Jz/1 -> Integrator/1, Mux3/2
  Add3/1 -> 1/Jz/1, Scope25/1
  Add1/1 -> Scope11/1, Add3/2
  ? -> Lf4/1
  Mux1/1 -> yaw rate/1
  w/1 -> Add/1
  w1/1 -> Add/2
  w/4/1 -> Add/3
  w/5/1 -> Add/4
  w/6/1 -> Add/5
  w/7/1 -> Add/6
  Mzfl/1 -> Add2/1
  Mzfr/1 -> Add2/2
  Add2/1 -> Scope10/1, Add3/3
  Mzrl/1 -> Add2/3
  Mzrr/1 -> Add2/4
  Lf4/1 -> Derivative/1, Integrator2/1, Mux1/1
  Mux3/1 -> yaw acc/1
  Derivative/1 -> Mux3/1
  Integrator2/1 -> Mux4/1
  Integrator3/1 -> Mux4/2
  Mux4/1 -> yaw/1

== system dof14model_rev/Subsys Handling/Subsystem ==
  u : Inport
  v : Inport  Port=2
  yaw angle : Inport  Port=3
  Add : Sum
  Add1 : Sum  Inputs=+-
  Integrator : Integrator
  Integrator1 : Integrator
  Product{,1..3} (4 alike) : Product  RndMeth=Zero
  X1 : Scope
  Y1 : Scope
  cos : Trigonometry  Operator=cos
  cos1 : Trigonometry
  X : Outport
  Y : Outport  Port=2
  wires:
  yaw angle/1 -> cos/1, cos1/1
  u/1 -> Product1/1, Product/1
  cos/1 -> Product1/2, Product3/2
  cos1/1 -> Product2/2, Product/2
  v/1 -> Product2/1, Product3/1
  Product1/1 -> Add1/1
  Product2/1 -> Add1/2
  Add1/1 -> Integrator/1
  Add/1 -> Integrator1/1
  Product3/1 -> Add/2
  Product/1 -> Add/1
  Integrator/1 -> X1/1, X/1
  Integrator1/1 -> Y1/1, Y/1

== system dof14model_rev/Subsys Tire/Subsys tfl ==
  S : Inport
  Fz : Inport  Port=2
  alpha : Inport  Port=3
  Gain1 : Gain  Gain=0.001
  Gain2 : Gain  Gain=180/pi
  Subsys Fx : Subsystem
  Subsys Fy : Subsystem
  Subsys Mz : Subsystem
  Fx : Outport
  Fy : Outport  Port=2
  Mz : Outport  Port=3
  wires:
  S/1 -> Subsys Fx/1(S)
  Fz/1 -> Gain1/1
  alpha/1 -> Gain2/1
  Subsys Fx/1(Fx) -> Fx/1
  Subsys Fy/1(Fy) -> Fy/1
  Subsys Mz/1(Mz) -> Mz/1
  Gain1/1 -> Subsys Fx/2(Fz), Subsys Fy/2(Fz), Subsys Mz/2(Fz)
  Gain2/1 -> Subsys Fy/1(alpha), Subsys Mz/1(alpha)

== system dof14model_rev/Subsys Tire/Subsys tfl1 ==
  S : Inport
  Fz : Inport  Port=2
  alpha : Inport  Port=3
  Gain1 : Gain  Gain=180/pi
  Gain2 : Gain  Gain=0.001
  Subsys Fx : Subsystem
  Subsys Fy : Subsystem
  Subsys Mz : Subsystem
  Fx : Outport
  Fy : Outport  Port=2
  Mz : Outport  Port=3
  wires:
  Subsys Fy/1(Fy) -> Fy/1
  Subsys Fx/1(Fx) -> Fx/1
  alpha/1 -> Gain1/1
  Fz/1 -> Gain2/1
  S/1 -> Subsys Fx/1(S)
  Subsys Mz/1(Mz) -> Mz/1
  Gain1/1 -> Subsys Mz/1(alpha), Subsys Fy/1(alpha)
  Gain2/1 -> Subsys Mz/2(Fz), Subsys Fy/2(Fz), Subsys Fx/2(Fz)

== system dof14model_rev/Subsys Tire/Subsys tfl2 ==
  S : Inport
  Fz : Inport  Port=2
  alpha : Inport  Port=3
  Gain1 : Gain  Gain=180/pi
  Gain2 : Gain  Gain=0.001
  Subsys Fx : Subsystem
  Subsys Fy : Subsystem
  Subsys Mz : Subsystem
  Fx : Outport
  Fy : Outport  Port=2
  Mz : Outport  Port=3
  wires:
  S/1 -> Subsys Fx/1(S)
  Fz/1 -> Gain2/1
  alpha/1 -> Gain1/1
  Subsys Fx/1(Fx) -> Fx/1
  Subsys Fy/1(Fy) -> Fy/1
  Subsys Mz/1(Mz) -> Mz/1
  Gain1/1 -> Subsys Fy/1(alpha), Subsys Mz/1(alpha)
  Gain2/1 -> Subsys Fx/2(Fz), Subsys Fy/2(Fz), Subsys Mz/2(Fz)

== system dof14model_rev/Subsys Tire/Subsys tfl3 ==
  S : Inport
  Fz : Inport  Port=2
  alpha : Inport  Port=3
  Gain : Gain  Gain=0.001
  Gain1 : Gain  Gain=180/pi
  Subsys Fx : Subsystem
  Subsys Fy : Subsystem
  Subsys Mz : Subsystem
  Fx : Outport
  Fy : Outport  Port=2
  Mz : Outport  Port=3
  wires:
  Subsys Mz/1(Mz) -> Mz/1
  Subsys Fy/1(Fy) -> Fy/1
  Subsys Fx/1(Fx) -> Fx/1
  alpha/1 -> Gain1/1
  Fz/1 -> Gain/1
  S/1 -> Subsys Fx/1(S)
  Gain1/1 -> Subsys Mz/1(alpha), Subsys Fy/1(alpha)
  Gain/1 -> Subsys Mz/2(Fz), Subsys Fy/2(Fz), Subsys Fx/2(Fz)

== system dof14model_rev/Subsys ride/Ffl ==
  Zufl dot : Inport
  Zsfl dot : Inport  Port=2
  Add : Sum
  Csfl : Gain  Gain=Csfl
  Integrator1 : Integrator
  Integrator2 : Integrator
  Ksfl : Gain  Gain=Ksfl
  Subtract : Sum  Inputs=+-
  Subtract1 : Sum  Inputs=+-
  Ffl : Outport
  wires:
  Zufl dot/1 -> Subtract/1, Integrator1/1
  Subtract/1 -> Csfl/1
  Zsfl dot/1 -> Subtract/2, Integrator2/1
  Subtract1/1 -> Ksfl/1
  Csfl/1 -> Add/1
  Ksfl/1 -> Add/2
  Add/1 -> Ffl/1
  Integrator1/1 -> Subtract1/1
  Integrator2/1 -> Subtract1/2

== system dof14model_rev/Subsys ride/Ffr ==
  Zufr dot : Inport
  Zsfr dot : Inport  Port=2
  Add : Sum
  Csfr : Gain  Gain=Csfr
  Integrator1 : Integrator
  Integrator2 : Integrator
  Ksfr : Gain  Gain=Ksfr
  Subtract : Sum  Inputs=+-
  Subtract1 : Sum  Inputs=+-
  Ffr : Outport
  wires:
  Add/1 -> Ffr/1
  Ksfr/1 -> Add/2
  Csfr/1 -> Add/1
  Subtract1/1 -> Ksfr/1
  Zsfr dot/1 -> Subtract/2, Integrator2/1
  Subtract/1 -> Csfr/1
  Zufr dot/1 -> Subtract/1, Integrator1/1
  Integrator1/1 -> Subtract1/1
  Integrator2/1 -> Subtract1/2

== system dof14model_rev/Subsys ride/Frl ==
  Zurl dot : Inport
  Zsrl dot : Inport  Port=2
  Add : Sum
  Csrl : Gain  Gain=Csrl
  Integrator1 : Integrator
  Integrator2 : Integrator
  Ksrl : Gain  Gain=Ksrl
  Subtract : Sum  Inputs=+-
  Subtract1 : Sum  Inputs=+-
  Frl : Outport
  wires:
  Zurl dot/1 -> Subtract/1, Integrator1/1
  Subtract/1 -> Csrl/1
  Zsrl dot/1 -> Subtract/2, Integrator2/1
  Subtract1/1 -> Ksrl/1
  Csrl/1 -> Add/1
  Ksrl/1 -> Add/2
  Add/1 -> Frl/1
  Integrator1/1 -> Subtract1/1
  Integrator2/1 -> Subtract1/2

== system dof14model_rev/Subsys ride/Frr ==
  Zurr dot : Inport
  Zsrr dot : Inport  Port=2
  Add : Sum
  Csrr : Gain  Gain=Csrr
  Integrator1 : Integrator
  Integrator2 : Integrator
  Ksrr : Gain  Gain=Ksrr
  Subtract : Sum  Inputs=+-
  Subtract1 : Sum  Inputs=+-
  Frr : Outport
  wires:
  Add/1 -> Frr/1
  Ksrr/1 -> Add/2
  Csrr/1 -> Add/1
  Subtract1/1 -> Ksrr/1
  Zsrr dot/1 -> Subtract/2, Integrator2/1
  Subtract/1 -> Csrr/1
  Zurr dot/1 -> Subtract/1, Integrator1/1
  Integrator1/1 -> Subtract1/1
  Integrator2/1 -> Subtract1/2

== system dof14model_rev/Subsys ride/Subsys Fz ==
  Ffl : Inport
  Ffr : Inport  Port=2
  Frl : Inport  Port=3
  Frr : Inport  Port=4
  Subsys Fzfl : Subsystem
  Subsys Fzfr : Subsystem
  Subsys Fzrl : Subsystem
  Subsys Fzrl1 : Subsystem
  To Workspace : ToWorkspace  VariableName=Fzfl1  SampleTime=-1
  To Workspace1 : ToWorkspace  VariableName=Fzfr1  SampleTime=-1
  To Workspace2 : ToWorkspace  VariableName=Fzrl1  SampleTime=-1
  To Workspace3 : ToWorkspace  VariableName=Fzrr1  SampleTime=-1
  Fzfl : Outport
  Fzfr : Outport  Port=2
  Fzrl : Outport  Port=3
  Fzrr : Outport  Port=4
  wires:
  Ffl/1 -> Subsys Fzfl/1(Ffl)
  Subsys Fzfl/1(Fzfl) -> Fzfl/1, To Workspace/1
  Ffr/1 -> Subsys Fzfr/1(Ffr)
  Subsys Fzfr/1(Fzfr) -> Fzfr/1, To Workspace1/1
  Frl/1 -> Subsys Fzrl/1(Frl)
  Subsys Fzrl/1(Fzrl) -> Fzrl/1, To Workspace2/1
  Frr/1 -> Subsys Fzrl1/1(Frr)
  Subsys Fzrl1/1(Fzrr) -> Fzrr/1, To Workspace3/1

== system dof14model_rev/Subsys ride/Subsys pitch ==
  Frl : Inport
  Frr : Inport  Port=2
  Ffl : Inport  Port=3
  Ffr : Inport  Port=4
  ax : Inport  Port=5
  1/Ip : Gain  Gain=1/Ip
  Ffl+Ffr : Sum
  Frl+Frr : Sum
  Integrator1 : Integrator
  Integrator2 : Integrator
  Scope1 : Scope
  Scope13 : Scope
  Subtract : Sum  Inputs=+-
  a : Gain  Gain=a
  b : Gain  Gain=b
  thita ddot : Outport
  wires:
  Frl+Frr/1 -> b/1
  Ffl+Ffr/1 -> a/1
  b/1 -> Subtract/1
  a/1 -> Subtract/2
  Frl/1 -> Frl+Frr/1
  Frr/1 -> Frl+Frr/2
  Ffl/1 -> Ffl+Ffr/1
  Ffr/1 -> Ffl+Ffr/2
  1/Ip/1 -> thita ddot/1, Integrator1/1
  Integrator1/1 -> Integrator2/1
  Integrator2/1 -> Scope13/1
  Subtract/1 -> 1/Ip/1
  ax/1 -> Scope1/1

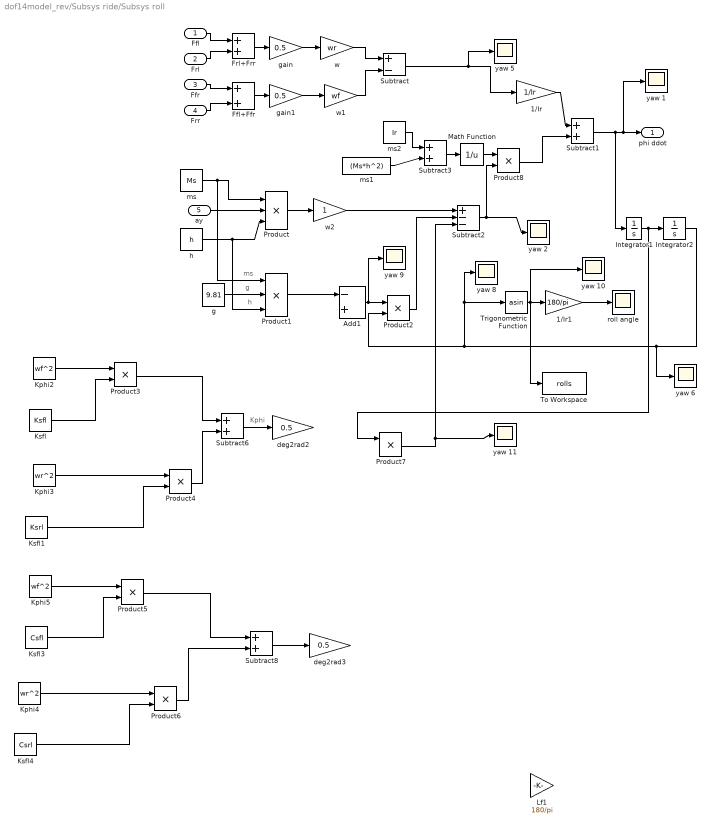
== system dof14model_rev/Subsys ride/Subsys roll ==
  note: g
  note: ms
  note: h
  note: Kphi
  Ffl : Inport
  Frl : Inport  Port=2
  Ffr : Inport  Port=3
  Frr : Inport  Port=4
  ay : Inport  Port=5
  1/Ir : Gain  Gain=1/Ir
  1/Ir1 : Gain  Gain=180/pi
  Add1 : Sum  Inputs=-+
  Ffl+Ffr : Sum
  Frl+Frr : Sum
  Integrator1 : Integrator
  Integrator2 : Integrator
  Kphi2 : Constant  Value=wf^2
  Kphi3 : Constant  Value=wr^2
  Kphi4 : Constant  Value=wr^2
  Kphi5 : Constant  Value=wf^2
  Ksfl : Constant  Value=Ksfl
  Ksfl1 : Constant  Value=Ksrl
  Ksfl3 : Constant  Value=Csfl
  Ksfl4 : Constant  Value=Csrl
  Lf1 : Gain  Gain=180/pi
  Math Function : Math  Operator=reciprocal  SignedPower=on
  Product : Product  Inputs=3  RndMeth=Zero
  Product1 : Product  Inputs=3  RndMeth=Zero
  Product{2..8} (7 alike) : Product  RndMeth=Zero
  Subtract : Sum  Inputs=+-
  Subtract{1,3,6,8} (4 alike) : Sum
  Subtract2 : Sum  Inputs=+--
  To Workspace : ToWorkspace  VariableName=rolls  SampleTime=-1
  Trigonometric Function : Trigonometry  Operator=asin
  deg2rad2 : Gain  Gain=0.5
  deg2rad3 : Gain  Gain=0.5
  g : Constant  Value=9.81
  gain : Gain  Gain=0.5
  gain1 : Gain  Gain=0.5
  h : Constant  Value=h
  ms : Constant  Value=Ms
  ms1 : Constant  Value=(Ms*h^2)
  ms2 : Constant  Value=Ir
  roll angle : Scope
  w : Gain  Gain=wr
  w1 : Gain  Gain=wf
  w2 : Gain
  yaw {1..2,5..6,8..11} (8 alike) : Scope
  phi ddot : Outport
  wires:
  Frr/1 -> Ffl+Ffr/2
  Ffr/1 -> Ffl+Ffr/1
  Frl/1 -> Frl+Frr/2
  Ffl/1 -> Frl+Frr/1
  Subtract/1 -> yaw 5/1, 1/Ir/1
  Ffl+Ffr/1 -> gain1/1
  Frl+Frr/1 -> gain/1
  gain/1 -> w/1
  gain1/1 -> w1/1
  w/1 -> Subtract/1
  w1/1 -> Subtract/2
  ms/1 -> Product/1, Product1/1
  h/1 -> Product/3, Product1/3
  g/1 -> Product1/2
  Product1/1 -> Add1/1
  Add1/1 -> Product2/1, yaw 9/1
  Product/1 -> w2/1
  ay/1 -> Product/2
  Subtract2/1 -> yaw 2/1, Product8/2
  Integrator1/1 -> Integrator2/1, Product7/1
  Product2/1 -> Subtract2/2
  Integrator2/1 -> Product2/2, Trigonometric Function/1, yaw 8/1, yaw 6/1
  Subtract1/1 -> phi ddot/1, yaw 1/1, Integrator1/1
  Trigonometric Function/1 -> 1/Ir1/1, yaw 10/1, To Workspace/1
  1/Ir1/1 -> roll angle/1
  Ksfl/1 -> Product3/2
  Kphi2/1 -> Product3/1
  Ksfl1/1 -> Product4/2
  Kphi3/1 -> Product4/1
  Ksfl3/1 -> Product5/2
  Kphi5/1 -> Product5/1
  Product3/1 -> Subtract6/1
  Product4/1 -> Subtract6/2
  Ksfl4/1 -> Product6/2
  Kphi4/1 -> Product6/1
  Product6/1 -> Subtract8/2
  Product5/1 -> Subtract8/1
  Subtract8/1 -> deg2rad3/1
  Product7/1 -> yaw 11/1, Subtract2/3
  Subtract6/1 -> deg2rad2/1
  ms2/1 -> Subtract3/1
  ms1/1 -> Subtract3/2
  1/Ir/1 -> Subtract1/1
  Subtract3/1 -> Math Function/1
  Product8/1 -> Subtract1/2
  Math Function/1 -> Product8/1
  w2/1 -> Subtract2/1

== system dof14model_rev/Subsys ride/Subsys sprung vertical ==
  Ffl : Inport
  Ffr : Inport  Port=2
  Frl : Inport  Port=3
  Frr : Inport  Port=4
  ay : Inport  Port=5
  Add : Sum  Inputs=+++++
  Gain : Gain  Gain=1/Ms
  Gain1 : Gain  Gain=Ms*h*2/wf
  Math Function1 : Math  Operator=square  SignedPower=on
  Zs ddot : Outport
  wires:
  Add/1 -> Gain/1
  Ffl/1 -> Add/1
  Ffr/1 -> Add/2
  Gain/1 -> Zs ddot/1
  Frl/1 -> Add/3
  Frr/1 -> Add/4
  ay/1 -> Gain1/1

== system dof14model_rev/Subsys ride/Subsys wheel fl ==
  Zufl : Inport
  Ffl : Inport  Port=2
  Zrfl : Inport  Port=3
  Divide : Product  Inputs=*/
  Ftfl : Subsystem
  Subtract : Sum  Inputs=+-
  mufl : Constant  Value=mufl
  Zufl ddot : Outport
  wires:
  Zrfl/1 -> Ftfl/1(Zrfl)
  Ftfl/1(Ftfl) -> Subtract/1
  Zufl/1 -> Ftfl/2(Zufl)
  Ffl/1 -> Subtract/2
  Subtract/1 -> Divide/1
  mufl/1 -> Divide/2
  Divide/1 -> Zufl ddot/1

== system dof14model_rev/Subsys ride/Subsys wheel fr ==
  Zufr : Inport
  Ffr : Inport  Port=2
  Zrfr : Inport  Port=3
  Divide : Product  Inputs=*/
  Ftfr : Subsystem
  Subtract1 : Sum  Inputs=+-
  mufr : Constant  Value=mufr
  Zufr ddot : Outport
  wires:
  Zrfr/1 -> Ftfr/1(Zrfr)
  Ftfr/1(Ftfr) -> Subtract1/1
  Zufr/1 -> Ftfr/2(Zufr)
  Ffr/1 -> Subtract1/2
  Subtract1/1 -> Divide/1
  mufr/1 -> Divide/2
  Divide/1 -> Zufr ddot/1

== system dof14model_rev/Subsys ride/Subsys wheel rl ==
  Zurl : Inport
  Frl : Inport  Port=2
  Zrrl : Inport  Port=3
  Divide : Product  Inputs=*/
  Ftrl : Subsystem
  Subtract2 : Sum  Inputs=+-
  murl : Constant  Value=murl
  Zurl ddot : Outport
  wires:
  Zrrl/1 -> Ftrl/1(Zrrl)
  Ftrl/1(Ftrl) -> Subtract2/1
  Zurl/1 -> Ftrl/2(Zurl)
  Frl/1 -> Subtract2/2
  Subtract2/1 -> Divide/1
  murl/1 -> Divide/2
  Divide/1 -> Zurl ddot/1

== system dof14model_rev/Subsys ride/Subsys wheel rr ==
  Zurr : Inport
  Frr : Inport  Port=2
  Zrrr : Inport  Port=3
  Divide : Product  Inputs=*/
  Ftfr2 : Subsystem
  Subtract3 : Sum  Inputs=+-
  murr : Constant  Value=murr
  Zurr ddot : Outport
  wires:
  Zrrr/1 -> Ftfr2/1(Zrrr)
  Ftfr2/1(Ftfr) -> Subtract3/1
  Zurr/1 -> Ftfr2/2(Zurr)
  Frr/1 -> Subtract3/2
  Subtract3/1 -> Divide/1
  murr/1 -> Divide/2
  Divide/1 -> Zurr ddot/1

== system dof14model_rev/Subsys ride/Zsfl dot ==
  Zs dot : Inport
  thita dot : Inport  Port=2
  chi dot : Inport  Port=3
  0.5 : Gain  Gain=0.5
  Add : Sum  Inputs=+-+
  a : Gain  Gain=a
  wfl : Gain  Gain=wf
  Zsfl dot : Outport
  wires:
  Zs dot/1 -> Add/1
  a/1 -> Add/2
  thita dot/1 -> a/1
  wfl/1 -> Add/3
  chi dot/1 -> 0.5/1
  Add/1 -> Zsfl dot/1
  0.5/1 -> wfl/1

== system dof14model_rev/Subsys ride/Zsfr dot ==
  Zs dot : Inport
  thita dot : Inport  Port=2
  chi dot : Inport  Port=3
  0.5 : Gain  Gain=0.5
  Add : Sum  Inputs=+--
  a : Gain  Gain=a
  w : Gain  Gain=wf
  Zsfr dot : Outport
  wires:
  Add/1 -> Zsfr dot/1
  chi dot/1 -> 0.5/1
  w/1 -> Add/3
  thita dot/1 -> a/1
  a/1 -> Add/2
  Zs dot/1 -> Add/1
  0.5/1 -> w/1

== system dof14model_rev/Subsys ride/Zsrl dot ==
  Zs dot : Inport
  thita dot : Inport  Port=2
  chi dot : Inport  Port=3
  0.5 : Gain  Gain=0.5
  Add : Sum  Inputs=+++
  b : Gain  Gain=b
  w : Gain  Gain=wr
  Zsrl dot : Outport
  wires:
  Zs dot/1 -> Add/1
  b/1 -> Add/2
  thita dot/1 -> b/1
  w/1 -> Add/3
  0.5/1 -> w/1
  chi dot/1 -> 0.5/1
  Add/1 -> Zsrl dot/1

== system dof14model_rev/Subsys ride/Zsrr dot ==
  Zs dot : Inport
  thita dot : Inport  Port=2
  chi dot : Inport  Port=3
  0.5 : Gain  Gain=0.5
  Add : Sum  Inputs=++-
  b : Gain  Gain=b
  w : Gain  Gain=wr
  Zsrr dot : Outport
  wires:
  Add/1 -> Zsrr dot/1
  chi dot/1 -> 0.5/1
  0.5/1 -> w/1
  w/1 -> Add/3
  thita dot/1 -> b/1
  b/1 -> Add/2
  Zs dot/1 -> Add/1

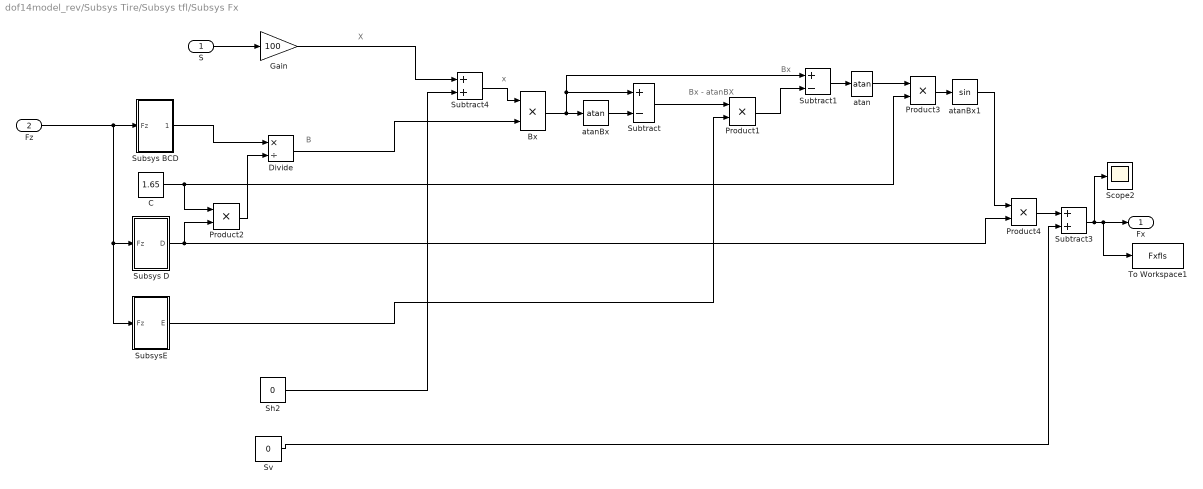
== system dof14model_rev/Subsys Tire/Subsys tfl/Subsys Fx ==
  note: B
  note: Bx
  note: Bx - atanBX
  note: X
  note: x
  S : Inport
  Fz : Inport  Port=2
  Bx : Product  RndMeth=Zero
  C : Constant  Value=1.65
  Divide : Product  Inputs=*/
  Gain : Gain  Gain=100
  Product{1..4} (4 alike) : Product  RndMeth=Zero
  Scope2 : Scope
  Sh2 : Constant  Value=0
  Subsys BCD : Subsystem
  Subsys D : Subsystem
  SubsysE : Subsystem
  Subtract : Sum  Inputs=+-
  Subtract1 : Sum  Inputs=+-
  Subtract3 : Sum
  Subtract4 : Sum
  Sv : Constant  Value=0
  To Workspace1 : ToWorkspace  VariableName=Fxfls  SampleTime=-1
  atan : Trigonometry  Operator=atan
  atanBx : Trigonometry  Operator=atan
  atanBx1 : Trigonometry
  Fx : Outport
  wires:
  C/1 -> Product2/1, Product3/2
  Subsys D/1(D) -> Product2/2, Product4/2
  Subsys BCD/1(BCD) -> Divide/1
  Product2/1 -> Divide/2
  Subtract3/1 -> Scope2/1, To Workspace1/1, Fx/1
  Product4/1 -> Subtract3/1
  Product3/1 -> atanBx1/1
  atanBx1/1 -> Product4/1
  atan/1 -> Product3/1
  S/1 -> Gain/1
  Subtract4/1 -> Bx/1
  Sv/1 -> Subtract3/2
  Subtract1/1 -> atan/1
  Product1/1 -> Subtract1/2
  SubsysE/1(E) -> Product1/2
  Subtract/1 -> Product1/1
  atanBx/1 -> Subtract/2
  Bx/1 -> Subtract/1, Subtract1/1, atanBx/1
  Divide/1 -> Bx/2
  Sh2/1 -> Subtract4/2
  Fz/1 -> Subsys BCD/1(Fz), Subsys D/1(Fz), SubsysE/1(Fz)
  Gain/1 -> Subtract4/1

== system dof14model_rev/Subsys Tire/Subsys tfl/Subsys Fy ==
  note: B
  note: Bx
  note: Bx - atanBX
  note: X
  note: x
  note: Sh
  alpha : Inport
  Fz : Inport  Port=2
  Bx : Product  RndMeth=Zero
  C : Constant  Value=1.3
  Divide : Product  Inputs=*/
  Product{1..4} (4 alike) : Product  RndMeth=Zero
  Scope2 : Scope
  Subsys BCD : Subsystem
  Subsys D : Subsystem
  SubsysE : Subsystem
  Subtract : Sum  Inputs=+-
  Subtract1 : Sum  Inputs=+-
  Subtract3 : Sum
  Subtract4 : Sum
  Sv : Constant  Value=0
  Sv1 : Constant  Value=0
  To Workspace1 : ToWorkspace  VariableName=Fyfls  SampleTime=-1
  atan : Trigonometry  Operator=atan
  atanBx : Trigonometry  Operator=atan
  atanBx1 : Trigonometry
  Fy : Outport
  wires:
  C/1 -> Product2/1, Product3/2
  Subsys D/1(D) -> Product2/2, Product4/2
  Product2/1 -> Divide/2
  Subtract3/1 -> To Workspace1/1, Fy/1, Scope2/1
  Product4/1 -> Subtract3/1
  Product3/1 -> atanBx1/1
  atanBx1/1 -> Product4/1
  atan/1 -> Product3/1
  Subtract4/1 -> Bx/1
  Sv/1 -> Subtract3/2
  Subtract1/1 -> atan/1
  Product1/1 -> Subtract1/2
  SubsysE/1(E) -> Product1/2
  Subtract/1 -> Product1/1
  atanBx/1 -> Subtract/2
  Bx/1 -> Subtract/1, Subtract1/1, atanBx/1
  Divide/1 -> Bx/2
  Sv1/1 -> Subtract4/2
  Subsys BCD/1(BCD) -> Divide/1
  alpha/1 -> Subtract4/1
  Fz/1 -> Subsys BCD/1(Fz), Subsys D/1(Fz), SubsysE/1(Fz)

== system dof14model_rev/Subsys Tire/Subsys tfl/Subsys Mz ==
  note: B
  note: Bx
  note: Bx - atanBX
  note: X
  note: x
  alpha : Inport
  Fz : Inport  Port=2
  Bx : Product  RndMeth=Zero
  C : Constant  Value=2.40
  Divide : Product  Inputs=*/
  Product{1..4} (4 alike) : Product  RndMeth=Zero
  Scope2 : Scope
  Sh2 : Constant  Value=0
  Subsys BCD : Subsystem
  Subsys D : Subsystem
  SubsysE : Subsystem
  Subtract : Sum  Inputs=+-
  Subtract1 : Sum  Inputs=+-
  Subtract3 : Sum
  Subtract4 : Sum
  Sv2 : Constant  Value=0
  To Workspace1 : ToWorkspace  VariableName=Mzfls  SampleTime=-1
  atan : Trigonometry  Operator=atan
  atanBx : Trigonometry  Operator=atan
  atanBx1 : Trigonometry
  Mz : Outport
  wires:
  C/1 -> Product2/1, Product3/2
  Subsys D/1(D) -> Product2/2, Product4/2
  Subsys BCD/1(BCD) -> Divide/1
  Product2/1 -> Divide/2
  Subtract3/1 -> Scope2/1, To Workspace1/1, Mz/1
  Product4/1 -> Subtract3/1
  Product3/1 -> atanBx1/1
  atanBx1/1 -> Product4/1
  atan/1 -> Product3/1
  alpha/1 -> Subtract4/1
  Subtract4/1 -> Bx/1
  Sv2/1 -> Subtract3/2
  Subtract1/1 -> atan/1
  Product1/1 -> Subtract1/2
  SubsysE/1(E) -> Product1/2
  Subtract/1 -> Product1/1
  atanBx/1 -> Subtract/2
  Bx/1 -> Subtract/1, Subtract1/1, atanBx/1
  Divide/1 -> Bx/2
  Sh2/1 -> Subtract4/2
  Fz/1 -> Subsys BCD/1(Fz), Subsys D/1(Fz), SubsysE/1(Fz)

== system dof14model_rev/Subsys Tire/Subsys tfl1/Subsys Fx ==
  note: x
  note: X
  note: Bx - atanBX
  note: Bx
  note: B
  S : Inport
  Fz : Inport  Port=2
  Bx : Product  RndMeth=Zero
  C : Constant  Value=1.65
  Divide : Product  Inputs=*/
  Gain : Gain  Gain=100
  Product{1..4} (4 alike) : Product  RndMeth=Zero
  Scope2 : Scope
  Sh2 : Constant  Value=0
  Subsys BCD : Subsystem
  Subsys D : Subsystem
  SubsysE : Subsystem
  Subtract : Sum  Inputs=+-
  Subtract1 : Sum  Inputs=+-
  Subtract3 : Sum
  Subtract4 : Sum
  Sv : Constant  Value=0
  To Workspace1 : ToWorkspace  VariableName=Fxfrs  SampleTime=-1
  atan : Trigonometry  Operator=atan
  atanBx : Trigonometry  Operator=atan
  atanBx1 : Trigonometry
  Fx : Outport
  wires:
  Gain/1 -> Subtract4/1
  Fz/1 -> SubsysE/1(Fz), Subsys D/1(Fz), Subsys BCD/1(Fz)
  Sh2/1 -> Subtract4/2
  Divide/1 -> Bx/2
  Bx/1 -> atanBx/1, Subtract1/1, Subtract/1
  atanBx/1 -> Subtract/2
  Subtract/1 -> Product1/1
  SubsysE/1(E) -> Product1/2
  Product1/1 -> Subtract1/2
  Subtract1/1 -> atan/1
  Sv/1 -> Subtract3/2
  Subtract4/1 -> Bx/1
  S/1 -> Gain/1
  atan/1 -> Product3/1
  atanBx1/1 -> Product4/1
  Product3/1 -> atanBx1/1
  Product4/1 -> Subtract3/1
  Subtract3/1 -> Fx/1, To Workspace1/1, Scope2/1
  Product2/1 -> Divide/2
  Subsys BCD/1(BCD) -> Divide/1
  Subsys D/1(D) -> Product4/2, Product2/2
  C/1 -> Product3/2, Product2/1
